simulink model "linear_engine_model"  (Simulink 8.1)
settings: Solver=VariableStepDiscrete  StartTime=0.0  StopTime=20  RelTol=1e-3
PreLoadFcn:
  | % engine model time step
  | Tm = 0.1;
  | 
  | % control time step
  | Tc = 0.5;
libraries: simulink x1
settings Model: Creator=jmahler  LastModifiedBy=jmahler
settings DataIOCC: SignalLoggingSaveFormat=Dataset
settings OptimizationCC: ExpressionDepthLimit=128
settings DebuggingCC: SolverPrmCheckMsg=none  FcnCallInpInsideContextMsg=EnableAllAsError
settings GRTTargetCC: CombineOutputUpdateFcns=on  GRTInterface=off

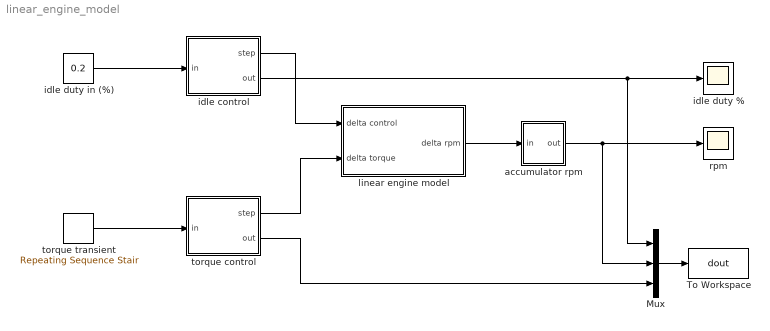
== system linear_engine_model ==
  Mux : Mux  Inputs=3
  To Workspace : ToWorkspace  VariableName=dout  SampleTime=-1  SaveFormat=Timeseries
  accumulator rpm : Subsystem  mask{T=Tm/2}
      mask prompts: T "Time Step"
  idle control : Subsystem  mask{T=Tm, S=1}
      mask prompts: T "Time Step"; S "Step Change (%)"
      mask Display:
      | disp('control')
      | port_label('input', 1, 'in')
      | port_label('output', 1, 'step')
      | port_label('output', 2, 'out')
  idle duty % : Scope
      settings: SaveName=ScopeData2
  idle duty in (%) : Constant  Value=0.2
  linear engine model : Subsystem  mask{T_L=0.1, Ts=Tm}
      mask prompts: T_L "Torque"; Ts "Sample Time (sec)"
      mask help: Linear Engine Model
      mask Display:
      | port_label('input', 1, '\Deltau(idle)', 'texmode', 'on')
      | port_label('input', 2, '\DeltaT_L(torque)', 'texmode', 'on')
      | port_label('output', 1, '\DeltaN (rpm)', 'texmode', 'on')
  rpm : Scope
  torque control : Subsystem  mask{T=Tm, S=10}
      mask prompts: T "Time Step"; S "Step Change (%)"
      mask Display:
      | disp('control')
      | port_label('input', 1, 'in')
      | port_label('output', 1, 'step')
      | port_label('output', 2, 'out')
  torque transient : simulink/Sources/Repeating Sequence Stair  OutValues=[0 10].'  tsamp=5  OutMin=[]  OutMax=[]  OutDataTypeStr=double  OutputDataTypeScalingMode=double  OutDataType=fixdt(0,8)  ConRadixGroup=Best Precision: Vector-wise  OutScaling=2^-12
  wires:
  linear engine model/1(delta rpm) -> accumulator rpm/1(in)
  accumulator rpm/1(out) -> Mux/2, rpm/1
  idle duty in (%)/1 -> idle control/1(in)
  torque control/1(step) -> linear engine model/2(delta torque)
  idle control/1(step) -> linear engine model/1(delta control)
  idle control/2(out) -> Mux/1, idle duty %/1
  torque transient/1 -> torque control/1(in)
  Mux/1 -> To Workspace/1
  torque control/2(out) -> Mux/3

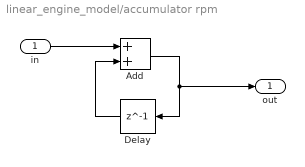
== system linear_engine_model/accumulator rpm ==
  in : Inport
  Add : Sum
  Delay : Delay  DelayLength=1
  out : Outport
  wires:
  in/1 -> Add/1
  Delay/1 -> Add/2
  Add/1 -> out/1, Delay/1

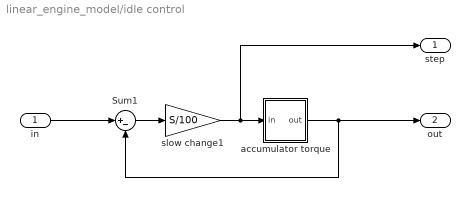
== system linear_engine_model/idle control ==
  in : Inport
  Sum1 : Sum  Inputs=|+-
  accumulator torque : Subsystem  mask{T=T}
      mask prompts: T "Time Step"
  slow change1 : Gain  Gain=S/100
  step : Outport
  out : Outport  Port=2
  wires:
  in/1 -> Sum1/1
  accumulator torque/1(out) -> Sum1/2, out/1
  Sum1/1 -> slow change1/1
  slow change1/1 -> step/1, accumulator torque/1(in)

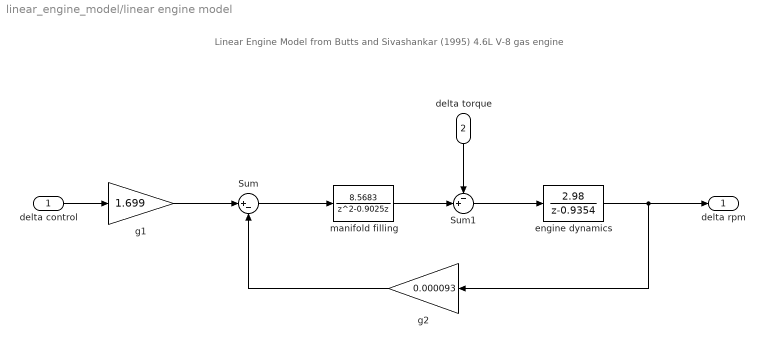
== system linear_engine_model/linear engine model ==
  note: Linear Engine Model
      | from Butts and Sivashankar (1995)
      | 4.6L V-8 gas engine
  delta control : Inport
  delta torque : Inport  Port=2
  Sum : Sum  Inputs=|+-
  Sum1 : Sum  Inputs=-+|
  engine dynamics : DiscreteTransferFcn  Numerator=[2.98]  Denominator=[1 -0.9354]  SampleTime=Ts
  g1 : Gain  Gain=1.699
  g2 : Gain  Gain=0.000093
  manifold filling : DiscreteTransferFcn  Numerator=[8.5683]  Denominator=[1 -0.9025 0]  SampleTime=Ts
  delta rpm : Outport
  wires:
  engine dynamics/1 -> delta rpm/1, g2/1
  delta control/1 -> g1/1
  Sum1/1 -> engine dynamics/1
  g2/1 -> Sum/2
  Sum/1 -> manifold filling/1
  g1/1 -> Sum/1
  manifold filling/1 -> Sum1/2
  delta torque/1 -> Sum1/1

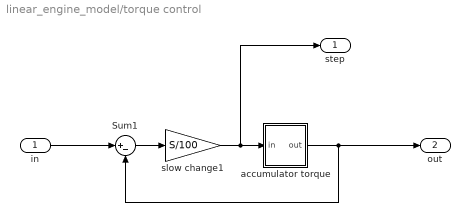
== system linear_engine_model/torque control ==
  in : Inport
  Sum1 : Sum  Inputs=|+-
  accumulator torque : Subsystem  mask{T=T}
      mask prompts: T "Time Step"
  slow change1 : Gain  Gain=S/100
  step : Outport
  out : Outport  Port=2
  wires:
  in/1 -> Sum1/1
  accumulator torque/1(out) -> Sum1/2, out/1
  Sum1/1 -> slow change1/1
  slow change1/1 -> step/1, accumulator torque/1(in)

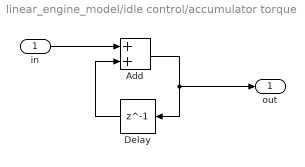
== system linear_engine_model/idle control/accumulator torque ==
  in : Inport
  Add : Sum
  Delay : Delay  DelayLength=1  SampleTime=T
  out : Outport
  wires:
  in/1 -> Add/1
  Delay/1 -> Add/2
  Add/1 -> out/1, Delay/1

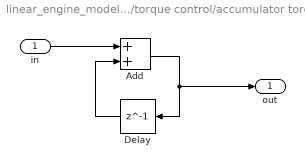
== system linear_engine_model/torque control/accumulator torque ==
  in : Inport
  Add : Sum
  Delay : Delay  DelayLength=1  SampleTime=T
  out : Outport
  wires:
  in/1 -> Add/1
  Delay/1 -> Add/2
  Add/1 -> out/1, Delay/1
